simulink model "data_ext"  (R2025b)
settings: Solver=ode4  StartTime=0.0  StopTime=5  FixedStep=0.01  RelTol=1e-3
undefined symbols (not defined in the file or in its folder): dspblkCoreblockFVToolHelper, gcbh
libraries: arduinolib x4
settings Model: ExtModeTrigDuration=2  Creator=sid  LastModifiedBy=sid
settings SolverCC: AutoInsertRateTranBlk=on
settings OptimizationCC: EnhancedBackFolding=on  PassReuseOutputArgsAs=Individual arguments  ZeroExternalMemoryAtStartup=off  ZeroInternalMemoryAtStartup=off  MaxStackSize=64  OptimizeBlockOrder=speed  DifferentSizesBufferReuse=on  OptimizationCustomize=off  EfficientTunableParamExpr=on
settings DebuggingCC: MultiTaskDSMMsg=none  ParameterTunabilityLossMsg=error
settings HardwareCC: ProdBitPerPointer=32.0  ProdBitPerSizeT=32.0  ProdBitPerPtrDiffT=32.0  ProdLargestAtomicInteger=Long  ProdLargestAtomicFloat=Double  ProdWordSize=32.0  ProdHWDeviceType=ARM Compatible->ARM Cortex  UseEmbeddedCoderFeatures=off
settings SFSimCC: MATLABDynamicMemAlloc=off
settings RTWCC: SystemTargetFile=ert.tlc  HardwareBoard=ESP32-WROOM (Arduino Compatible)  TLCOptions="-aInlineSetEventsForThisBaseRateFcn=TLC_FALSE -aSuppressMultiTaskScheduler=TLC_FALSE  -aRateBasedStepFcn=0"  TemplateMakefile=ert_default_tmf  Toolchain=ESP32  Description=Embedded Coder
settings CodeAppCC: ForceParamTrailComments=on  IgnoreCustomStorageClasses=off  OperatorAnnotations=on  SimulinkDataObjDesc=on  SFDataObjDesc=on  InsertBlockDesc=on
settings ERTTargetCC: ExtModeTransport=3.0  ExtModeStaticAlloc=on  ExtModeAutomaticAllocSize=off  ExtModeStaticAllocSize=65536.0  ExtModeMexFile=ext_xcp  ExtModeIntrfLevel=Level2 - Open  InlinedParameterPlacement=Hierarchical  SupportContinuousTime=on  SupportNonInlinedSFcns=on  SupportVariableSizeSignals=on

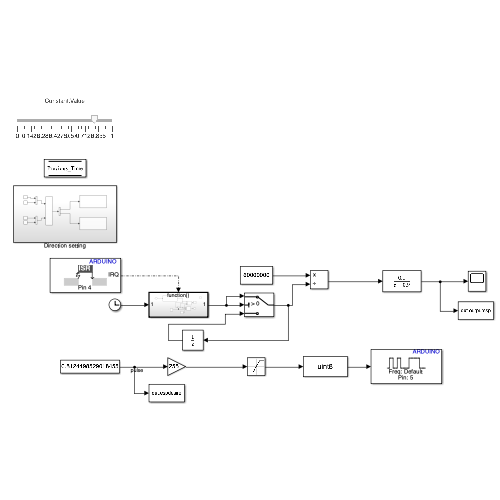
[thumbnail: Simulink's stored preview of the top-level diagram]
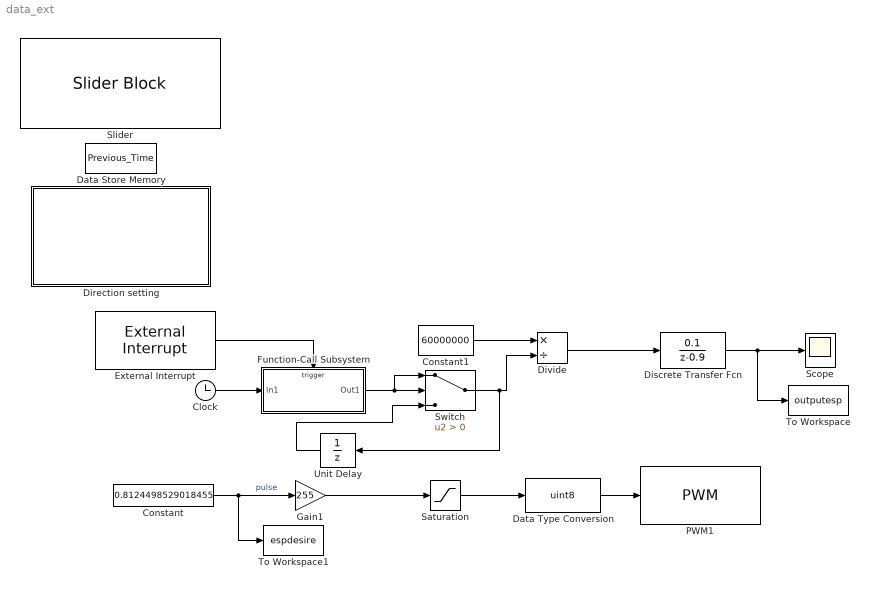
== system data_ext ==
  Clock : Clock
  Constant : Constant  Value=0.8124498529018455  OutMin=0  OutMax=1
  Constant1 : Constant  Value=60000000
  Data Store Memory : DataStoreMemory  DataStoreName=Previous_Time  WriteAfterWriteMsg=warning  ShowAdditionalParam=off  OutDataTypeStr=uint32
  Data Type Conversion : DataTypeConversion  OutDataTypeStr=uint8  SaturateOnIntegerOverflow=off  RndMeth=Floor
  Direction setting : Subsystem
  Discrete Transfer Fcn : DiscreteTransferFcn  LoadFcn=dspblkCoreblockFVToolHelper(gcbh,'load');  Numerator=[0.1]  Denominator=[1 -0.9]
      settings: CopyFcn=dspblkCoreblockFVToolHelper(gcbh,'copy');  DeleteFcn=dspblkCoreblockFVToolHelper(gcbh,'close');  ModelCloseFcn=dspblkCoreblockFVToolHelper(gcbh,'close');  PreSaveFcn=dspblkCoreblockFVToolHelper(gcbh,'presave');  PostSaveFcn=dspblkCoreblockFVToolHelper(gcbh,'postsave');  CloseFcn=dspblkCoreblockFVToolHelper(gcbh,'close');
  Divide : Product  Inputs=*/
  External Interrupt : arduinolib/External Interrupt  Pin=4  PullUp=off  Mode=RISING  InterruptSimulationInput=off
  Function-Call Subsystem : Subsystem  TreatAsAtomicUnit=on
  Gain1 : Gain  Gain=255
  PWM1 : arduinolib/PWM  pinNumber=5  frequencyType=Default  desiredFrequency=490.2  achievableFrequency=490.2
  Saturation : Saturate  UpperLimit=255  LowerLimit=0
  Scope : Scope
      settings: ActiveDisplayYMinimum=-3423.6258318427854  ActiveDisplayYMaximum=30812.632486585077
  Slider : SliderBlock  ScaleMax=1
  Switch : Switch  Criteria=u2 > Threshold  SaturateOnIntegerOverflow=off  InputSameDT=off
  To Workspace : ToWorkspace  VariableName=outputesp  SaveFormat=Timeseries  SampleTime=-1
  To Workspace1 : ToWorkspace  VariableName=espdesire  SaveFormat=Timeseries  SampleTime=-1
  Unit Delay : UnitDelay  InitialCondition=60000000  SampleTime=-1  HasFrameUpgradeWarning=on
  wires:
  Constant1/1 -> Divide/1
  Discrete Transfer Fcn/1 -> To Workspace/1, Scope/1
  Constant/1 -> Gain1/1, To Workspace1/1  "pulse"
  Data Type Conversion/1 -> PWM1/1
  Switch/1 -> Divide/2, Unit Delay/1
  Divide/1 -> Discrete Transfer Fcn/1
  Clock/1 -> Function-Call Subsystem/1(In1)
  Gain1/1 -> Saturation/1
  Unit Delay/1 -> Switch/3
  Saturation/1 -> Data Type Conversion/1
  Function-Call Subsystem/1(Out1) -> Switch/1, Switch/2
  External Interrupt/1 -> Function-Call Subsystem/Trigger

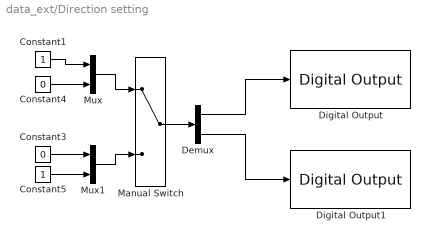
== system data_ext/Direction setting ==
  Constant1 : Constant  OutMin=0  OutMax=1  OutDataTypeStr=uint8
  Constant3 : Constant  Value=0  OutMin=0  OutMax=1  OutDataTypeStr=uint8
  Constant4 : Constant  Value=0  OutMin=0  OutMax=1  OutDataTypeStr=uint8
  Constant5 : Constant  OutMin=0  OutMax=1  OutDataTypeStr=uint8
  Demux : Demux  Outputs=2
  Digital Output : arduinolib/Digital Output  pinNumber=19  Direction=output  blockPlatform=arduino
  Digital Output1 : arduinolib/Digital Output  pinNumber=21  Direction=output  blockPlatform=arduino
  Manual Switch : ManualSwitch
  Mux : Mux  Inputs=2
  Mux1 : Mux  Inputs=2
  wires:
  Constant4/1 -> Mux/2
  Mux1/1 -> Manual Switch/2
  Demux/1 -> Digital Output/1
  Demux/2 -> Digital Output1/1
  Constant1/1 -> Mux/1
  Mux/1 -> Manual Switch/1
  Constant5/1 -> Mux1/2
  Constant3/1 -> Mux1/1
  Manual Switch/1 -> Demux/1

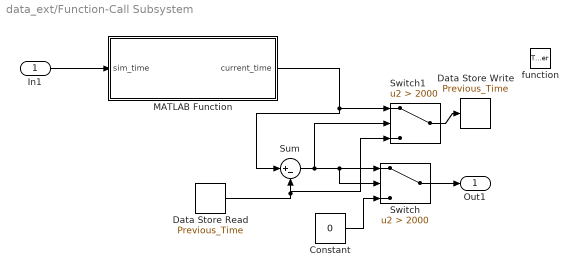
== system data_ext/Function-Call Subsystem ==
  In1 : Inport
  function : TriggerPort  TriggerType=function-call  VariantControl=(inherit)
  Constant : Constant  Value=0
  Data Store Read : DataStoreRead  Priority=1  DataStoreName=Previous_Time  IndexOptions=Index vector (dialog)  Indices=1  OutputSizes=1
  Data Store Write : DataStoreWrite  Priority=10  DataStoreName=Previous_Time  IndexOptions=Index vector (dialog)  Indices=1  OutputSizes=1
  MATLAB Function : MATLAB Function  TreatAsAtomicUnit=on
  Sum : Sum  Inputs=|+-
  Switch : Switch  Criteria=u2 > Threshold  Threshold=2000  SaturateOnIntegerOverflow=off  InputSameDT=off
  Switch1 : Switch  Criteria=u2 > Threshold  Threshold=2000  SaturateOnIntegerOverflow=off  InputSameDT=off
  Out1 : Outport
  wires:
  Data Store Read/1 -> Switch1/3, Sum/2
  MATLAB Function/1(current_time) -> Switch1/1, Sum/1
  In1/1 -> MATLAB Function/1(sim_time)
  Sum/1 -> Switch1/2, Switch/2, Switch/1
  Switch/1 -> Out1/1
  Constant/1 -> Switch/3
  Switch1/1 -> Data Store Write/1

== matlab function data_ext/Function-Call Subsystem/MATLAB Function ==
  data: current_time output; sim_time input
function current_time = get_micros(sim_time)
    current_time = uint32(0); 
    
    if coder.target('rtw')
        % --- HARDWARE MODE (ESP32) ---
        % Call the C function 'micros()' directly
        current_time = coder.ceval('micros'); 
        
    else
        % --- SIMULATION MODE (Computer) ---
        % Convert the Simulation Time (seconds) to Microseconds
        % 1 second = 1,000,000 microseconds
        current_time = uint32(sim_time * 1000000);
    end
end
